simulink model "FINALBCM_Team5"  (R2018b)
settings: Solver=VariableStepAuto  SolverName=FixedStepAuto  StartTime=0.0  StopTime=4.0  RelTol=1e-3
undefined symbols (not defined in the file): sigbuilder_block
libraries: simulink x20
settings Model: Creator=99003181  LastModifiedBy=99003181
settings DataIOCC: ReturnWorkspaceOutputs=on
settings OptimizationCC: OptimizeBlockIOStorage=off  OptimizeDataStoreBuffers=off  BusAssignmentInplaceUpdate=off
settings DebuggingCC: SFUnexpectedBacktrackingDiag=warning  SFNoUnconditionalDefaultTransitionDiag=warning
settings RTWCC: GenerateReport=on  BuildConfiguration=Debug  LaunchReport=on
settings CodeAppCC: ForceParamTrailComments=on  MATLABSourceComments=on  EnableCustomComments=on
settings GRTTargetCC: CombineSignalStateStructs=on  SupportVariableSizeSignals=on  MultiInstanceErrorCode=Warning
settings ConfigComp: CovEnable=on  RecordCoverage=on  CovModelRefEnable=on

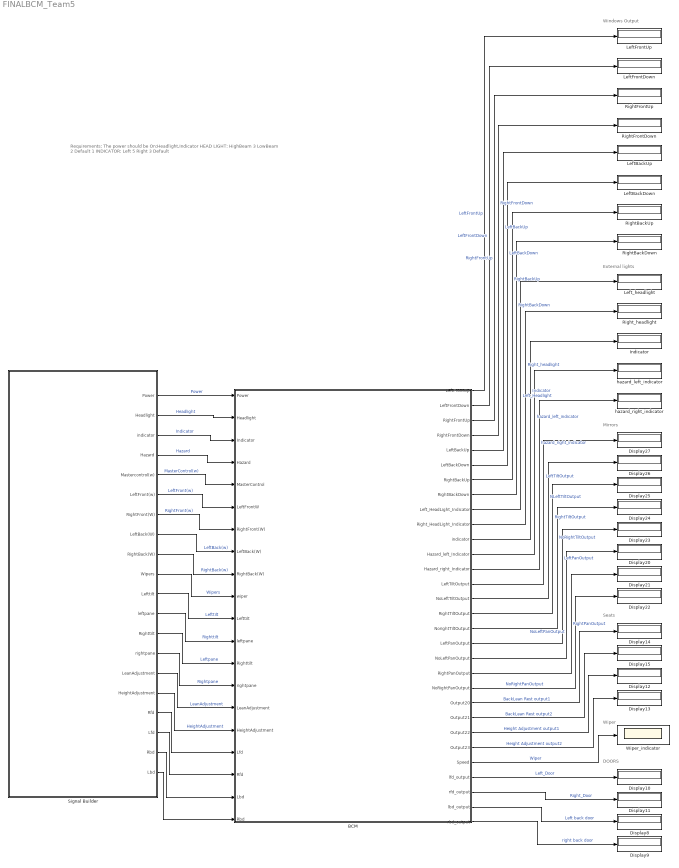
== system FINALBCM_Team5 ==
  note: Requirements:
      | The power should be On:Headlight,Indicator
      | HEAD LIGHT:
      | HighBeam	3
      | LowBeam	2
      | Default		1
      |
      | INDICATOR:
      | Left			5
      | Right 		3
      | Default
  note: Windows Output
  note: Wiper
  note: External lights
  note: Seats
  note: Mirrors
  note: DOORS
  BCM : Subsystem
  Display{8..15,20..27} (16 alike) : Display
  Indicator : Display
  LeftBackDown : Display
  LeftBackUp : Display
  LeftFrontDown : Display
  LeftFrontUp : Display
  Left_headlight : Display
  RightBackDown : Display
  RightBackUp : Display
  RightFrontDown : Display
  RightFrontUp : Display
  Right_headlight : Display
  Signal Builder : Subsystem  Tag=STV Subsys  LoadFcn=sigbuilder_block('load');  StartFcn=sigbuilder_block('start');  StopFcn=sigbuilder_block('stop');  ClipboardFcn=sigbuilder_block('clipboard');  mask(Sigbuilder block){tuvar=[0:10]}
      mask help: Simulink:masks:SigbuilderBlock_MD
      mask init:
      | if ~strcmp(get_param(bdroot(gcbh),'SimulationStatus'),'stopped') tuvar = sigbuilder_block('maskInit'); end
      settings: CopyFcn=sigbuilder_block('copy');  DeleteFcn=sigbuilder_block('delete');  ModelCloseFcn=sigbuilder_block('modelClose');  PreSaveFcn=sigbuilder_block('preSave');  PauseFcn=sigbuilder_block('pause');  ContinueFcn=sigbuilder_block('continue');  NameChangeFcn=sigbuilder_block('namechange');  OpenFcn=sigbuilder_block('open',[7.5 30.75 1011 481.5 ]);  CloseFcn=sigbuilder_block('close');
      mask Display: plot(0, 0, 100, 100,[2, 2, 32, 32, 2], [68, 8, 8, 68, 68],[32, 2], [38, 38], [32, 19, 2],[53, 60, 44], [32, 17, 17, 2],[16, 16, 31, 31]);txt = getActiveGroup(gcbh);text(2, 100, txt,'verticalAlignment', 'top');
  Wiper_indicator : Scope
  hazard_left_indicator : Display
  hazard_right_indicator : Display
  wires:
  Signal Builder/5(Mastercontrol(w)) -> BCM/5(MasterControl)  "MasterControl(w)"
  Signal Builder/8(LeftBack(W)) -> BCM/8(LeftBack(W))  "LeftBack(w)"
  Signal Builder/16(HeightAdjustment) -> BCM/16(HeightAdjustment)  "HeightAdjustment"
  Signal Builder/19(Rbd) -> BCM/19(Lbd)
  Signal Builder/11(Lefttilt) -> BCM/11(Lefttilt)  "Lefttilt"
  Signal Builder/20(Lbd) -> BCM/20(Rbd)
  Signal Builder/4(Hazard) -> BCM/4(Hazard)  "Hazard"
  Signal Builder/15(LeanAdjustment) -> BCM/15(LeanAdjustment)  "LeanAdjustment"
  Signal Builder/9(RightBack(W)) -> BCM/9(RightBack(W))  "RightBack(w)"
  Signal Builder/10(Wipers) -> BCM/10(wiper)  "Wipers"
  Signal Builder/6(LeftFront(w)) -> BCM/6(LeftFrontW)  "LeftFront(w)"
  Signal Builder/12(leftpane) -> BCM/12(leftpane)  "Righttilt"
  Signal Builder/1(Power) -> BCM/1(Power)  "Power"
  Signal Builder/7(RightFront(W)) -> BCM/7(RightFront(W))  "RightFront(w)"
  Signal Builder/14(rightpane) -> BCM/14(rightpane)  "Rightpane"
  Signal Builder/13(Righttilt) -> BCM/13(Righttilt)  "Leftpane"
  Signal Builder/2(Headlight) -> BCM/2(Headlight)  "Headlight"
  Signal Builder/17(Rfd) -> BCM/17(Lfd)
  Signal Builder/3(indicator) -> BCM/3(Indicator)  "Indicator"
  Signal Builder/18(Lfd) -> BCM/18(Rfd)
  BCM/21(NoRightPanOutput) -> Display22/1  "NoRightPanOutput"
  BCM/4(RightFrontDown) -> RightFrontDown/1  "RightFrontDown"
  BCM/12(Hazard_left_Indicator) -> hazard_left_indicator/1  "hazard_left_indicator"
  BCM/15(NoLeftTiltOutput) -> Display26/1  "NLeftTiltOutput"
  BCM/25(Output23) -> Display13/1  "Height Adjustment output2"
  BCM/26(Speed) -> Wiper_indicator/1  "Wiper"
  BCM/20(RightPanOutput) -> Display21/1  "RightPanOutput"
  BCM/1(LeftFrontUp) -> LeftFrontUp/1  "LeftFrontUp"
  BCM/24(Output22) -> Display12/1  "Height Adjustment output1"
  BCM/2(LeftFrontDown) -> LeftFrontDown/1  "LeftFrontDown"
  BCM/14(LeftTiltOutput) -> Display27/1  "LeftTiltOutput"
  BCM/10(Right_HeadLight_Indicator) -> Right_headlight/1  "Right_headlight"
  BCM/22(Output20) -> Display14/1  "BackLean Rest output1"
  BCM/7(RightBackUp) -> RightBackUp/1  "RightBackUp"
  BCM/23(Output21) -> Display15/1  "BackLean Rest output2"
  BCM/6(LeftBackDown) -> LeftBackDown/1  "LeftBackDown"
  BCM/16(RightTiltOutput) -> Display25/1  "RightTiltOutput"
  BCM/3(RightFrontUp) -> RightFrontUp/1  "RightFrontUp"
  BCM/5(LeftBackUp) -> LeftBackUp/1  "LeftBackUp"
  BCM/17(NorightTiltOutput) -> Display24/1  "NoRightTiltOutput"
  BCM/8(RightBackDown) -> RightBackDown/1  "RightBackDown"
  BCM/18(LeftPanOutput) -> Display23/1  "LeftPanOutput"
  BCM/29(lbd_output) -> Display8/1  "Left back door"
  BCM/19(NoLeftPanOutput) -> Display20/1  "NoLeftPanOutput"
  BCM/27(lfd_output) -> Display10/1  "Left_Door"
  BCM/9(Left_HeadLight_Indicator) -> Left_headlight/1  "Left_Headlight"
  BCM/30(rbd_output) -> Display9/1  "right back door"
  BCM/11(indicator) -> Indicator/1  "Indicator"
  BCM/28(rfd_output) -> Display11/1  "Right_Door"
  BCM/13(Hazard_right_Indicator) -> hazard_right_indicator/1  "hazard_right_indicator"

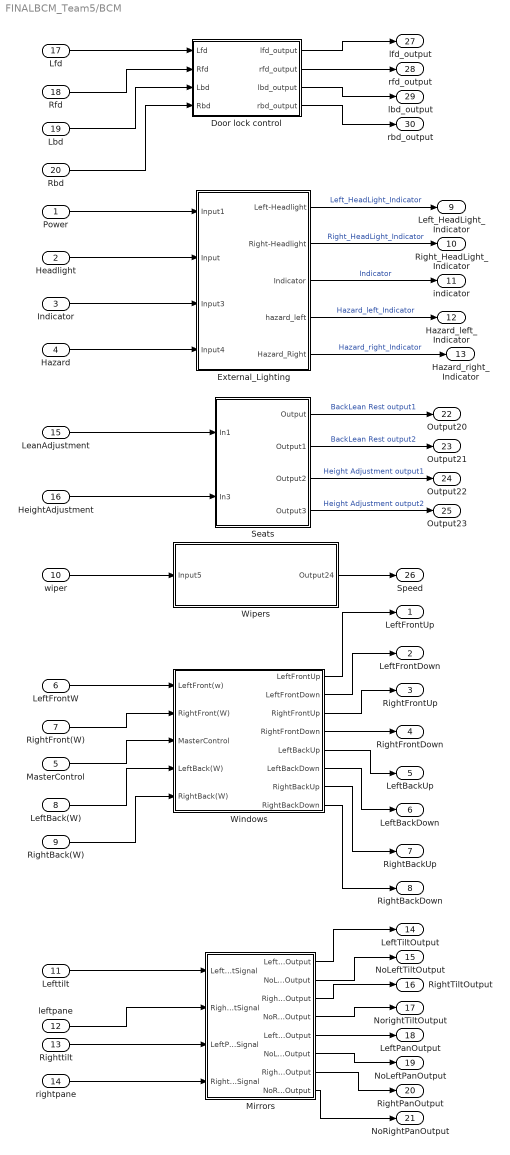
== system FINALBCM_Team5/BCM ==
  Power : Inport
  Headlight : Inport  Port=2
  Indicator : Inport  Port=3
  Hazard : Inport  Port=4
  MasterControl : Inport  Port=5
  LeftFrontW : Inport  Port=6
  RightFront(W) : Inport  Port=7
  LeftBack(W) : Inport  Port=8
  RightBack(W) : Inport  Port=9
  wiper : Inport  Port=10
  Lefttilt : Inport  Port=11
  leftpane : Inport  Port=12
  Righttilt : Inport  Port=13
  rightpane : Inport  Port=14
  LeanAdjustment : Inport  Port=15
  HeightAdjustment : Inport  Port=16
  Lfd : Inport  Port=17
  Rfd : Inport  Port=18
  Lbd : Inport  Port=19
  Rbd : Inport  Port=20
  Door lock control : Subsystem
  External_Lighting : Subsystem
  Mirrors : Subsystem
  Seats : Subsystem
  Windows : Subsystem
  Wipers : Subsystem
  LeftFrontUp : Outport
  LeftFrontDown : Outport  Port=2
  RightFrontUp : Outport  Port=3
  RightFrontDown : Outport  Port=4
  LeftBackUp : Outport  Port=5
  LeftBackDown : Outport  Port=6
  RightBackUp : Outport  Port=7
  RightBackDown : Outport  Port=8
  Left_HeadLight_Indicator : Outport  Port=9
  Right_HeadLight_Indicator : Outport  Port=10
  indicator : Outport  Port=11
  Hazard_left_Indicator : Outport  Port=12
  Hazard_right_Indicator : Outport  Port=13
  LeftTiltOutput : Outport  Port=14
  NoLeftTiltOutput : Outport  Port=15
  RightTiltOutput : Outport  Port=16
  NorightTiltOutput : Outport  Port=17
  LeftPanOutput : Outport  Port=18
  NoLeftPanOutput : Outport  Port=19
  RightPanOutput : Outport  Port=20
  NoRightPanOutput : Outport  Port=21
  Output20 : Outport  Port=22
  Output21 : Outport  Port=23
  Output22 : Outport  Port=24
  Output23 : Outport  Port=25
  Speed : Outport  Port=26
  lfd_output : Outport  Port=27
  rfd_output : Outport  Port=28
  lbd_output : Outport  Port=29
  rbd_output : Outport  Port=30
  wires:
  Seats/4("Output3 ") -> Output23/1  "Height Adjustment output2"
  LeftBack(W)/1 -> Windows/4(LeftBack(W))
  External_Lighting/5(Hazard_Right) -> Hazard_right_Indicator/1  "Hazard_right_Indicator"
  leftpane/1 -> Mirrors/2(RightTiltSignal)
  Windows/1(LeftFrontUp) -> LeftFrontUp/1
  Seats/3("Output2 ") -> Output22/1  "Height Adjustment output1"
  Windows/2(LeftFrontDown) -> LeftFrontDown/1
  wiper/1 -> Wipers/1(Input5)
  Windows/8(RightBackDown) -> RightBackDown/1
  External_Lighting/1(Left-Headlight) -> Left_HeadLight_Indicator/1  "Left_HeadLight_Indicator"
  Windows/4(RightFrontDown) -> RightFrontDown/1
  Hazard/1 -> External_Lighting/4(Input4)
  Windows/7(RightBackUp) -> RightBackUp/1
  External_Lighting/4(hazard_left) -> Hazard_left_Indicator/1  "Hazard_left_Indicator"
  Windows/3(RightFrontUp) -> RightFrontUp/1
  Windows/5(LeftBackUp) -> LeftBackUp/1
  Windows/6(LeftBackDown) -> LeftBackDown/1
  Indicator/1 -> External_Lighting/3(Input3)
  RightBack(W)/1 -> Windows/5(RightBack(W))
  Headlight/1 -> External_Lighting/2(Input)
  MasterControl/1 -> Windows/3(MasterControl)
  RightFront(W)/1 -> Windows/2(RightFront(W))
  LeftFrontW/1 -> Windows/1(LeftFront(w))
  Rfd/1 -> Door lock control/2(Rfd)
  Rbd/1 -> Door lock control/4(Rbd)
  Lbd/1 -> Door lock control/3(Lbd)
  Door lock control/4(rbd_output) -> rbd_output/1
  Door lock control/3(lbd_output) -> lbd_output/1
  Door lock control/2(rfd_output) -> rfd_output/1
  Door lock control/1(lfd_output) -> lfd_output/1
  Lfd/1 -> Door lock control/1(Lfd)
  LeanAdjustment/1 -> Seats/1("In1 ")
  Wipers/1(Output24) -> Speed/1
  External_Lighting/2(Right-Headlight) -> Right_HeadLight_Indicator/1  "Right_HeadLight_Indicator"
  Seats/1("Output ") -> Output20/1  "BackLean Rest output1"
  External_Lighting/3(Indicator) -> indicator/1  "Indicator"
  Seats/2("Output1 ") -> Output21/1  "BackLean Rest output2"
  Power/1 -> External_Lighting/1(Input1)
  HeightAdjustment/1 -> Seats/2("In3 ")
  Lefttilt/1 -> Mirrors/1(LeftTiltSignal)
  Mirrors/8(NoRightPanOutput) -> NoRightPanOutput/1
  Mirrors/7(RightPanOutput) -> RightPanOutput/1
  Mirrors/6(NoLeftPanOutput) -> NoLeftPanOutput/1
  Mirrors/5(LeftPanOutput) -> LeftPanOutput/1
  Mirrors/4(NoRightTiltOutput) -> NorightTiltOutput/1
  Mirrors/3(RightTiltOutput) -> RightTiltOutput/1
  Mirrors/2(NoLeftTiltOutput) -> NoLeftTiltOutput/1
  Mirrors/1(LeftTiltOutput) -> LeftTiltOutput/1
  rightpane/1 -> Mirrors/4(RightPanSignal)
  Righttilt/1 -> Mirrors/3(LeftPanSignal)

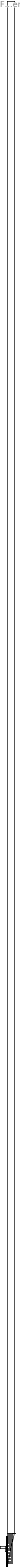
== system FINALBCM_Team5/Signal Builder ==
  Demux : Demux  Tag=STV Demux  Outputs=20
      settings: DisplayOption=none
  FromWs : FromWorkspace  Tag=STV FromWs  VariableName=tuvar
      SigBuilderData=|
      | common.afterFinalStr = 'Extrapolate'
      | common.sampleTime = 0
      | dataSet.timeRange = [0 10]
      | dataSet.name = 'Group 1'
      | sbobj.Groups.Name = 'Group 1'
      | sbobj.Groups.Signals(1).Name = 'Power'
      | sbobj.Groups.Signals(1).XData = [0 0.5 0.5 1 1 1.5 1.5 2 2 2.5 2.5 3 3 3.5 3.5 4 4.5 5 5 5.5 5.5 6 6 6.5 6.5 7 7 7.5 7.5 8 8 8.5 8.5 9 9 9.5 10]
      | sbobj.Groups.Signals(1).YData = [0.995 0.995 0 0 1 1 0 0 0.98 0.98 0 0 1 1 0 0 0 0 1 1 0 0 1 1 0 0 0.005 0.005 0 0 0.99 0.99 1 1 0 0 0]
      | sbobj.Groups.Signals(2).Name = 'Headlight'
      | sbobj.Groups.Signals(2).XData = [0 0.5 0.5 1 1 1.5 1.5 2 2 2.5 2.5 3 3 3.5 3.5 4 4 4.5 4.5 5 5 5.5 5.5 6 6 6.5 6.5 7 7 7.5 7.5 8 8 8.5 8.5 9 9 9.5 9.5 10]
      | sbobj.Groups.Signals(2).YData = [3 3 0 0 2 2 0 0 1.02 1.02 0 0 1.02 1.02 0 0 2 2 0 0 2.98 2.98 0 0 2 2 0 0 2.96 2.96 0 0 2 2 0 0 0.98 0.98 0 0]
      | sbobj.Groups.Signals(3).Name = 'indicator'
      | sbobj.Groups.Signals(3).XData = [0 0.5 0.5 1 1 1.5 1.5 2 2 2.5 2.5 3 3 3.5 3.5 4 4 4.5 4.5 5 5 5.5 5.5 6 6 6.5 6.5 7 7 7.5 7.5 8 8 8.5 8.5 9 9 9.5 9.5 10]
      | sbobj.Groups.Signals(3).YData = [5 5 0 0 0.98 0.98 0 0 3 3 0 0 5 5 0 0 3 3 0 0 2 2 0 0 1.02 1.02 0 0 1 1 0 0 -0.02 -0.02 0 0 3 3 0 0]
      | sbobj.Groups.Signals(4).Name = 'Hazard'
      | sbobj.Groups.Signals(4).XData = [0 0.5 0.5 1 1 1.5 1.5 2 2 2.5 2.5 3 3 3.5 3.5 4 4 4.5 4.5 5 5 5.5 5.5 6 6 6.5 6.5 7 7 7.5 7.5 8 8 8.5 8.5 9 9 9.5 9.5 10]
      | sbobj.Groups.Signals(4).YData = [2 2 0 0 2 2 0 0 2 2 0 0 2 2 0 0 2 2 0 0 2 2 0 0 2 2 0 0 2 2 0 0 2 2 0 0 2 2 0 0]
      | sbobj.Groups.Signals(5).Name = 'Mastercontrol(w)'
      | sbobj.Groups.Signals(5).XData = [0 1.25 1.25 6 6 9.92 9.92 10]
      | sbobj.Groups.Signals(5).YData = [0 0 1.05 1.05 0.75 0.75 0 0]
      | sbobj.Groups.Signals(6).Name = 'LeftFront(w)'
      | sbobj.Groups.Signals(6).XData = [0 2 2 3.8 3.8 10]
      | sbobj.Groups.Signals(6).YData = [0 0 1 1 -1 -1]
      | sbobj.Groups.Signals(7).Name = 'RightFront(W)'
      | sbobj.Groups.Signals(7).XData = [0 3.82 3.82 5.39 5.39 8 8 10]
      | sbobj.Groups.Signals(7).YData = [0 0 1 1 -1 -1 0.6 0.6]
      | sbobj.Groups.Signals(8).Name = 'LeftBack(W)'
      | sbobj.Groups.Signals(8).XData = [0 5.43 5.43 7.02 7.02 10]
      | sbobj.Groups.Signals(8).YData = [0 0 1 1 -1 -1]
      | sbobj.Groups.Signals(9).Name = 'RightBack(W)'
      | sbobj.Groups.Signals(9).XData = [0 7.06 7.06 8.92 8.92 10]
      | sbobj.Groups.Signals(9).YData = [0 0 1 1 -1 -1]
      | sbobj.Groups.Signals(10).Name = 'Wipers'
      | sbobj.Groups.Signals(10).XData = [0 1 1 2 2 3 3 4 4 5 5 6 6 7 7 8 8 9 9 10]
      | sbobj.Groups.Signals(10).YData = [0.2 0.2 0.4 0.4 0.6 0.6 0.2 0.2 0.4 0.4 0.6 0.6 0.2 0.2 0.4 0.4 0.6 0.6 0.2 0.2]
      | sbobj.Groups.Signals(11).Name = 'Lefttilt'
      | sbobj.Groups.Signals(11).XData = [0 3.86 3.86 5.71 5.71 10]
      | sbobj.Groups.Signals(11).YData = [0 0 1 1 0 0]
      | sbobj.Groups.Signals(12).Name = 'leftpane'
      | sbobj.Groups.Signals(12).XData = [0 2 2 3.8 3.8 10]
      | sbobj.Groups.Signals(12).YData = [0 0 1 1 0 0]
      | sbobj.Groups.Signals(13).Name = 'Righttilt'
      | sbobj.Groups.Signals(13).XData = [0 5.86 5.86 7.58 7.58 10]
      | sbobj.Groups.Signals(13).YData = [0 0 1 1 0 0]
      | sbobj.Groups.Signals(14).Name = 'rightpane'
      | sbobj.Groups.Signals(14).XData = [0 7.87 7.87 9.78 9.78 10]
      | sbobj.Groups.Signals(14).YData = [0 0 1 1 0 0]
      | sbobj.Groups.Signals(15).Name = 'LeanAdjustment'
      | sbobj.Groups.Signals(15).XData = [0 3.82 3.82 5.39 5.39 8 8 10]
      | sbobj.Groups.Signals(15).YData = [0 0 1 1 -1 -1 0.6 0.6]
      | sbobj.Groups.Signals(16).Name = 'HeightAdjustment'
      | sbobj.Groups.Signals(16).XData = [0 5.43 5.43 7.02 7.02 10]
      | sbobj.Groups.Signals(16).YData = [0 0 1 1 -1 -1]
      | sbobj.Groups.Signals(17).Name = 'Rfd'
      | sbobj.Groups.Signals(17).XData = [0 5 5 10]
      | sbobj.Groups.Signals(17).YData = [0 0 1 1]
      | sbobj.Groups.Signals(18).Name = 'Lfd'
      | sbobj.Groups.Signals(18).XData = [0 5 5 10]
      | sbobj.Groups.Signals(18).YData = [0 0 1 1]
      | sbobj.Groups.Signals(19).Name = 'Rbd'
      | sbobj.Groups.Signals(19).XData = [0 5 5 10]
      | sbobj.Groups.Signals(19).YData = [0 0 1 1]
      | sbobj.Groups.Signals(20).Name = 'Lbd'
      | sbobj.Groups.Signals(20).XData = [0 5 5 10]
      | sbobj.Groups.Signals(20).YData = [0 0 1 1]
  Power : Outport  Tag=STV Outport  VectorParamsAs1DForOutWhenUnconnected=off
  Headlight : Outport  Tag=STV Outport  Port=2  VectorParamsAs1DForOutWhenUnconnected=off
  indicator : Outport  Tag=STV Outport  Port=3  VectorParamsAs1DForOutWhenUnconnected=off
  Hazard : Outport  Tag=STV Outport  Port=4  VectorParamsAs1DForOutWhenUnconnected=off
  Mastercontrol(w) : Outport  Tag=STV Outport  Port=5
  LeftFront(w) : Outport  Tag=STV Outport  Port=6
  RightFront(W) : Outport  Tag=STV Outport  Port=7
  LeftBack(W) : Outport  Tag=STV Outport  Port=8
  RightBack(W) : Outport  Tag=STV Outport  Port=9
  Wipers : Outport  Tag=STV Outport  Port=10
  Lefttilt : Outport  Tag=STV Outport  Port=11
  leftpane : Outport  Tag=STV Outport  Port=12
  Righttilt : Outport  Tag=STV Outport  Port=13
  rightpane : Outport  Tag=STV Outport  Port=14
  LeanAdjustment : Outport  Tag=STV Outport  Port=15
  HeightAdjustment : Outport  Tag=STV Outport  Port=16
  Rfd : Outport  Tag=STV Outport  Port=17
  Lfd : Outport  Tag=STV Outport  Port=18
  Rbd : Outport  Tag=STV Outport  Port=19
  Lbd : Outport  Tag=STV Outport  Port=20
  wires:
  FromWs/1 -> Demux/1
  Demux/1 -> Power/1
  Demux/2 -> Headlight/1
  Demux/3 -> indicator/1
  Demux/4 -> Hazard/1
  Demux/5 -> Mastercontrol(w)/1
  Demux/6 -> LeftFront(w)/1
  Demux/7 -> RightFront(W)/1
  Demux/8 -> LeftBack(W)/1
  Demux/9 -> RightBack(W)/1
  Demux/10 -> Wipers/1
  Demux/11 -> Lefttilt/1
  Demux/12 -> leftpane/1
  Demux/13 -> Righttilt/1
  Demux/14 -> rightpane/1
  Demux/15 -> LeanAdjustment/1
  Demux/16 -> HeightAdjustment/1
  Demux/17 -> Rfd/1
  Demux/18 -> Lfd/1
  Demux/19 -> Rbd/1
  Demux/20 -> Lbd/1

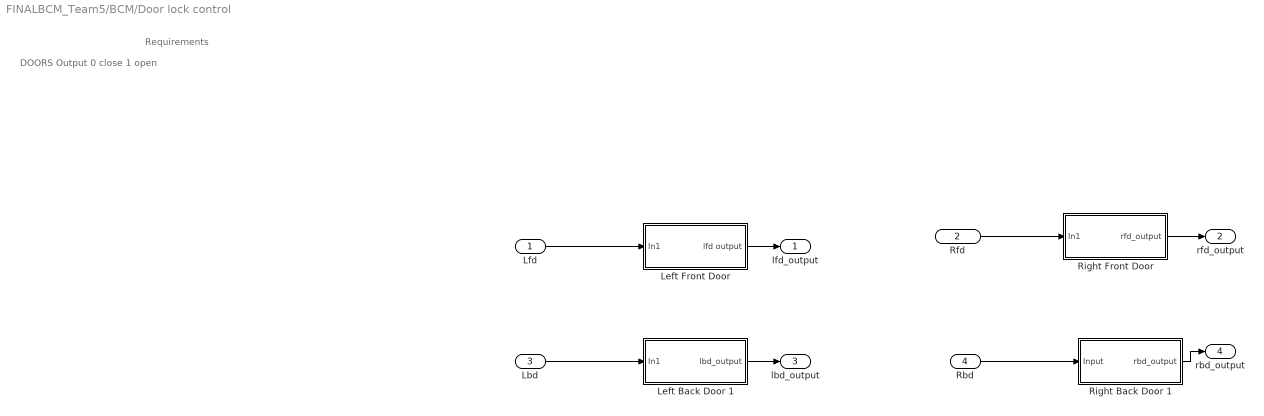
== system FINALBCM_Team5/BCM/Door lock control ==
  note: DOORS
      | Output
      |
      | 0
      | close
      |
      | 1
      | open
  note: Requirements
  Lfd : Inport
  Rfd : Inport  Port=2
  Lbd : Inport  Port=3
  Rbd : Inport  Port=4
  Left Back Door 1 : Subsystem
  "Left Front Door " : Subsystem
  Right Back Door 1 : Subsystem
  "Right Front Door " : Subsystem
  lfd_output : Outport
  rfd_output : Outport  Port=2
  lbd_output : Outport  Port=3
  rbd_output : Outport  Port=4
  wires:
  Lfd/1 -> "Left Front Door "/1(In1)
  "Left Front Door "/1(lfd output) -> lfd_output/1
  Rfd/1 -> "Right Front Door "/1(In1)
  "Right Front Door "/1(rfd_output) -> rfd_output/1
  Lbd/1 -> Left Back Door 1/1(In1)
  Left Back Door 1/1(lbd_output) -> lbd_output/1
  Rbd/1 -> Right Back Door 1/1(Input)
  Right Back Door 1/1(rbd_output) -> rbd_output/1

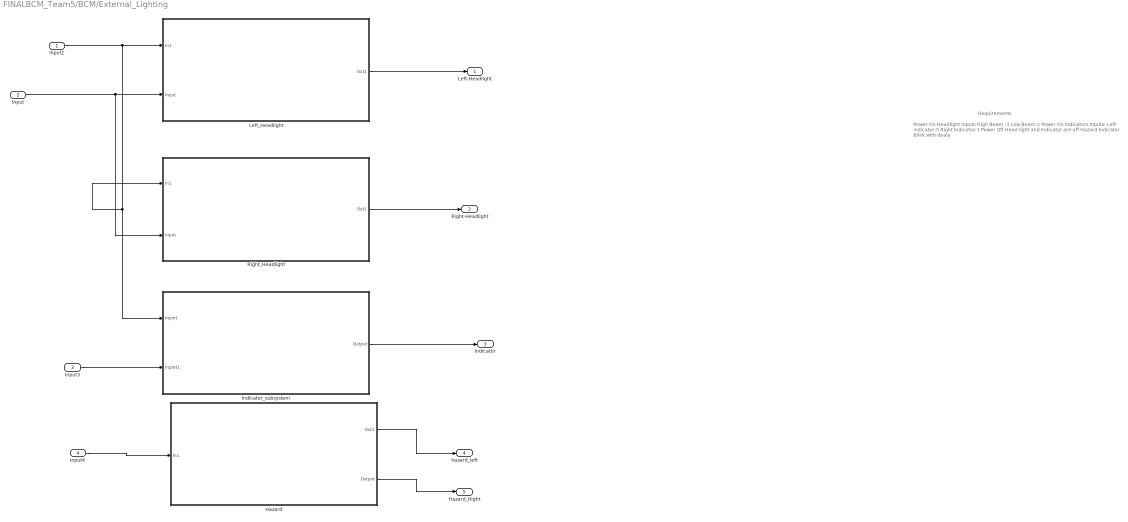
== system FINALBCM_Team5/BCM/External_Lighting ==
  note: Requirements
  note: Power
      | On
      | Headlight Inputs
      | High Beam :3
      | Low Beam:2
      |
      | Power On
      | Indicators Inputs:
      | Left indicator:5
      | Right Indicator:3
      |
      | Power Off
      | Head light and Indicator are off
      |
      | Hazard Indicator
      | Blink with dealy
  Input1 : Inport
  Input : Inport  Port=2
  Input3 : Inport  Port=3
  Input4 : Inport  Port=4
  Hazard : Subsystem
  Indicator_subsystem : Subsystem
  Left_Headlight : Subsystem
  Right_Headlight : Subsystem
  Left-Headlight : Outport  VectorParamsAs1DForOutWhenUnconnected=off
  Right-Headlight : Outport  Port=2  VectorParamsAs1DForOutWhenUnconnected=off
  Indicator : Outport  Port=3  VectorParamsAs1DForOutWhenUnconnected=off
  hazard_left : Outport  Port=4  VectorParamsAs1DForOutWhenUnconnected=off
  Hazard_Right : Outport  Port=5
  wires:
  Input1/1 -> Left_Headlight/1(In1), Indicator_subsystem/1(Inport), Right_Headlight/1(In1)
  Left_Headlight/1(Out1) -> Left-Headlight/1
  Right_Headlight/1(Out1) -> Right-Headlight/1
  Hazard/1(Out1) -> hazard_left/1
  Input4/1 -> Hazard/1(In1)
  Input/1 -> Right_Headlight/2(Input), Left_Headlight/2(Input)
  Indicator_subsystem/1(Output) -> Indicator/1
  Input3/1 -> Indicator_subsystem/2(Inport1)
  Hazard/2(Output) -> Hazard_Right/1

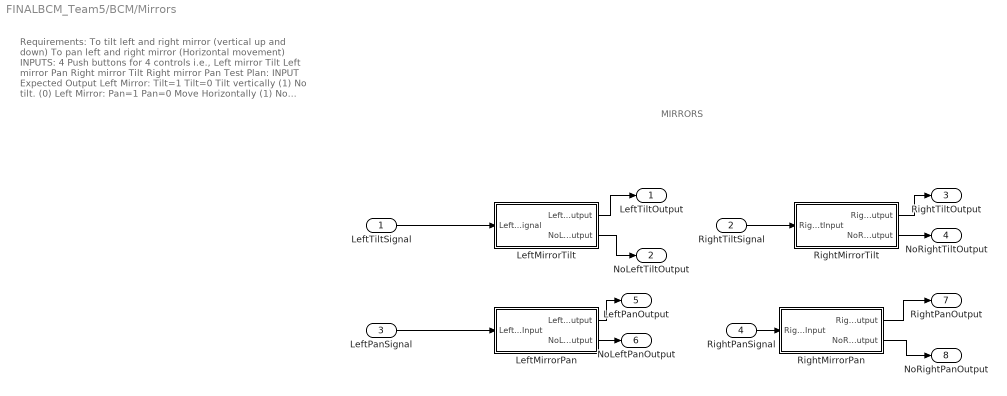
== system FINALBCM_Team5/BCM/Mirrors ==
  note: MIRRORS
  note: Requirements:
      | To tilt left and right mirror (vertical up and down)
      | To pan left and right mirror (Horizontal movement)
      | INPUTS:
      | 4 Push buttons for 4 controls i.e.,
      | Left mirror Tilt
      | Left mirror Pan
      | Right mirror Tilt
      | Right mirror Pan
      | Test Plan:
      |
      | INPUT
      | Expected Output
      |
      | Left Mirror: Tilt=1
      | Tilt=0
      | Tilt vertically (1)
      | No tilt. (0)
      |
      | Left Mirror: Pan=1
      | Pan=0
      | Move Horizontally (1)
      | No movement. (0)
      |
      | Right Mirror: Tilt=1
      | Tilt=0
      | Tilt vertically (1)
      | No tilt. (0)
      |
      | Right Mirror: Pan=1
      | Pan=0
      | Move Horizontally(1)
      | No movement.(0)
  LeftTiltSignal : Inport
  RightTiltSignal : Inport  Port=2
  LeftPanSignal : Inport  Port=3
  RightPanSignal : Inport  Port=4
  LeftMirrorPan : Subsystem
  "LeftMirrorTilt " : Subsystem
  RightMirrorPan : Subsystem
  "RightMirrorTilt " : Subsystem
  LeftTiltOutput : Outport
  NoLeftTiltOutput : Outport  Port=2
  RightTiltOutput : Outport  Port=3
  NoRightTiltOutput : Outport  Port=4
  LeftPanOutput : Outport  Port=5
  NoLeftPanOutput : Outport  Port=6
  RightPanOutput : Outport  Port=7
  NoRightPanOutput : Outport  Port=8
  wires:
  RightPanSignal/1 -> RightMirrorPan/1(RightPanInput)
  "RightMirrorTilt "/2(NoRightTiltOutput) -> NoRightTiltOutput/1
  LeftPanSignal/1 -> LeftMirrorPan/1(LeftPanInput)
  "RightMirrorTilt "/1(RightTiltOutput) -> RightTiltOutput/1
  "LeftMirrorTilt "/1(LeftTiltOutput) -> LeftTiltOutput/1
  LeftTiltSignal/1 -> "LeftMirrorTilt "/1(LeftTiltSignal)
  RightTiltSignal/1 -> "RightMirrorTilt "/1(RightTiltInput)
  LeftMirrorPan/1(LeftPanOutput) -> LeftPanOutput/1
  RightMirrorPan/1(RightPanOutput) -> RightPanOutput/1
  RightMirrorPan/2(NoRightPanOutput) -> NoRightPanOutput/1
  LeftMirrorPan/2(NoLeftPanOutput) -> NoLeftPanOutput/1
  "LeftMirrorTilt "/2(NoLeftTiltOutput) -> NoLeftTiltOutput/1

== system FINALBCM_Team5/BCM/Seats ==
  note: Requirements
      | Input
      | Output
      |
      | BackrestLean
      | 1
      | 0
      | -1
      | Invalid
      | Off
      | On
      |
      | Seatheight Adjustment
      | 1
      | 0
      | -1
      | On
      | Off
      | Invalid
  "In1 " : Inport
  "In3 " : Inport  Port=2
  BackrestLean : Subsystem
  SeatheightAdjustment : Subsystem
  "Output " : Outport
  "Output1 " : Outport  Port=2
  "Output2 " : Outport  Port=3
  "Output3 " : Outport  Port=4
  wires:
  BackrestLean/1("Output ") -> "Output "/1  "BackLean output"
  "In3 "/1 -> SeatheightAdjustment/1("In1 ")  "height input"
  SeatheightAdjustment/2("Output1 ") -> "Output3 "/1  "height output 2"
  SeatheightAdjustment/1("Output ") -> "Output2 "/1  "height Output 1"
  BackrestLean/2("Output1 ") -> "Output1 "/1  "BackLean output"
  "In1 "/1 -> BackrestLean/1("In1 ")  "BackLean Input"

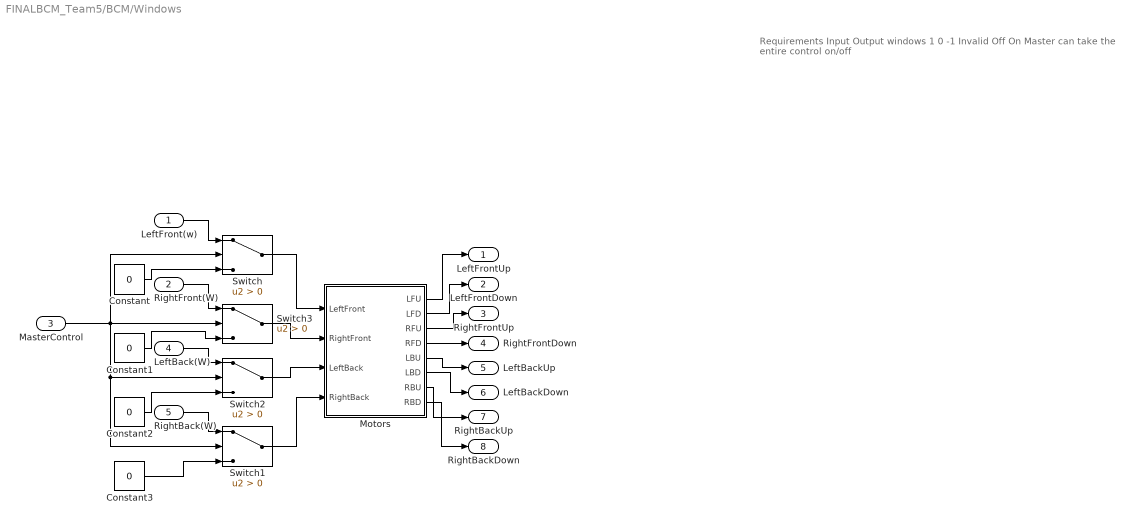
== system FINALBCM_Team5/BCM/Windows ==
  note: Requirements
      | Input
      | Output
      |
      | windows
      | 1
      | 0
      | -1
      | Invalid
      | Off
      | On
      |
      | Master
      | can take the entire control
      | on/off
  LeftFront(w) : Inport
  RightFront(W) : Inport  Port=2
  MasterControl : Inport  Port=3
  LeftBack(W) : Inport  Port=4
  RightBack(W) : Inport  Port=5
  Constant{,1..3} (4 alike) : Constant  Value=0
  Motors : Subsystem
  Switch{,1..3} (4 alike) : Switch  Criteria=u2 > Threshold
  LeftFrontUp : Outport
  LeftFrontDown : Outport  Port=2
  RightFrontUp : Outport  Port=3
  RightFrontDown : Outport  Port=4
  LeftBackUp : Outport  Port=5
  LeftBackDown : Outport  Port=6
  RightBackUp : Outport  Port=7
  RightBackDown : Outport  Port=8
  wires:
  MasterControl/1 -> Switch3/2, Switch/2, Switch1/2, Switch2/2
  Constant3/1 -> Switch1/3
  LeftBack(W)/1 -> Switch2/1
  Motors/1(LFU) -> LeftFrontUp/1
  Switch/1 -> Motors/1(LeftFront)
  LeftFront(w)/1 -> Switch/1
  Constant/1 -> Switch/3
  Switch1/1 -> Motors/4(RightBack)
  Constant2/1 -> Switch2/3
  Switch3/1 -> Motors/2(RightFront)
  Constant1/1 -> Switch3/3
  RightBack(W)/1 -> Switch1/1
  RightFront(W)/1 -> Switch3/1
  Motors/6(LBD) -> LeftBackDown/1
  Switch2/1 -> Motors/3(LeftBack)
  Motors/5(LBU) -> LeftBackUp/1
  Motors/2(LFD) -> LeftFrontDown/1
  Motors/3(RFU) -> RightFrontUp/1
  Motors/7(RBU) -> RightBackUp/1
  Motors/8(RBD) -> RightBackDown/1
  Motors/4(RFD) -> RightFrontDown/1

== system FINALBCM_Team5/BCM/Wipers ==
  note: Inputs (Sensor Input)
      | Output Speed
      |
      | Value < 10
      | Low Speed
      |
      | Value <=30
      | Mid Speed
      |
      | Value <=50
      | High Speed
      |
      | Value >50
      | Very High Speed
  Input5 : Inport
  Enable Subsystem : Subsystem  TreatAsAtomicUnit=on
  Ignition : Constant
  Subsystem : Subsystem
  scaling_factor : Gain  Gain=50
  Output24 : Outport
  wires:
  Ignition/1 -> Enable Subsystem/Enable
  Enable Subsystem/1(Out1) -> Subsystem/1(In1)
  scaling_factor/1 -> Enable Subsystem/1(In1)
  Input5/1 -> scaling_factor/1
  Subsystem/1(Out1) -> Output24/1

== system FINALBCM_Team5/BCM/Door lock control/Left Back Door 1 ==
  In1 : Inport
  Constant : Constant  Value=0
  Ramp : simulink/Sources/Ramp  slope=0  start=0  InitialOutput=1
  Switch : Switch  Criteria=u2 > Threshold
  lbd_output : Outport
  wires:
  In1/1 -> Switch/2
  Switch/1 -> lbd_output/1
  Constant/1 -> Switch/3
  Ramp/1 -> Switch/1

== system FINALBCM_Team5/BCM/Door lock control/Left Front Door  ==
  In1 : Inport
  Constant : Constant  Value=0
  Ramp : simulink/Sources/Ramp  slope=0  start=0  InitialOutput=1
  S1 : Switch  Criteria=u2 > Threshold
  lfd output : Outport
  wires:
  In1/1 -> S1/2
  S1/1 -> lfd output/1
  Constant/1 -> S1/3
  Ramp/1 -> S1/1

== system FINALBCM_Team5/BCM/Door lock control/Right Back Door 1 ==
  Input : Inport
  Constant : Constant  Value=0
  Ramp_input : simulink/Sources/Ramp  slope=0  start=0  InitialOutput=1
  Switch : Switch  Criteria=u2 > Threshold
  rbd_output : Outport
  wires:
  Input/1 -> Switch/2
  Switch/1 -> rbd_output/1
  Constant/1 -> Switch/3
  Ramp_input/1 -> Switch/1

== system FINALBCM_Team5/BCM/Door lock control/Right Front Door  ==
  In1 : Inport
  Constant : Constant  Value=0
  Ramp : simulink/Sources/Ramp  slope=0  start=0  InitialOutput=1
  Switch : Switch  Criteria=u2 > Threshold
  rfd_output : Outport
  wires:
  In1/1 -> Switch/2
  Switch/1 -> rfd_output/1
  Constant/1 -> Switch/3
  Ramp/1 -> Switch/1

== system FINALBCM_Team5/BCM/External_Lighting/Hazard ==
  In1 : Inport
  AND2 : Logic  IconShape=distinctive  AllPortsSameDT=off  OutDataTypeStr=boolean
  Enable_Input : DiscretePulseGenerator  PulseType=Time based  Period=1  PulseWidth=50
  Triggered Subsystem : Subsystem  TreatAsAtomicUnit=on
  Out1 : Outport  VectorParamsAs1DForOutWhenUnconnected=off
  Output : Outport  Port=2
  wires:
  Triggered Subsystem/1(Output) -> Output/1, Out1/1
  In1/1 -> AND2/2
  AND2/1 -> Triggered Subsystem/1(In1)
  Enable_Input/1 -> AND2/1, Triggered Subsystem/Trigger

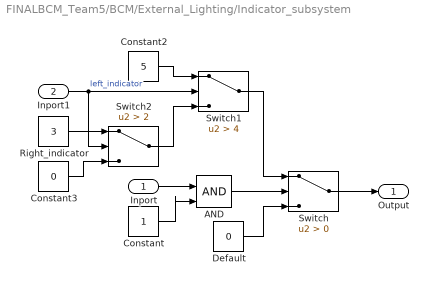
== system FINALBCM_Team5/BCM/External_Lighting/Indicator_subsystem ==
  Inport : Inport
  Inport1 : Inport  Port=2
  AND : Logic  IconShape=distinctive  AllPortsSameDT=off  OutDataTypeStr=boolean
  Constant : Constant
  Constant2 : Constant  Value=5
  Constant3 : Constant  Value=0
  Default : Constant  Value=0
  Right_indicator : Constant  Value=3
  Switch : Switch  Criteria=u2 > Threshold
  Switch1 : Switch  Criteria=u2 > Threshold  Threshold=4
  Switch2 : Switch  Criteria=u2 > Threshold  Threshold=2
  Output : Outport  VectorParamsAs1DForOutWhenUnconnected=off
  wires:
  Inport/1 -> AND/1
  Switch/1 -> Output/1
  Constant/1 -> AND/2
  Constant2/1 -> Switch1/1
  Default/1 -> Switch/3
  Switch1/1 -> Switch/1
  AND/1 -> Switch/2
  Right_indicator/1 -> Switch2/1
  Constant3/1 -> Switch2/3
  Switch2/1 -> Switch1/3
  Inport1/1 -> Switch2/2, Switch1/2  "left_indicator"

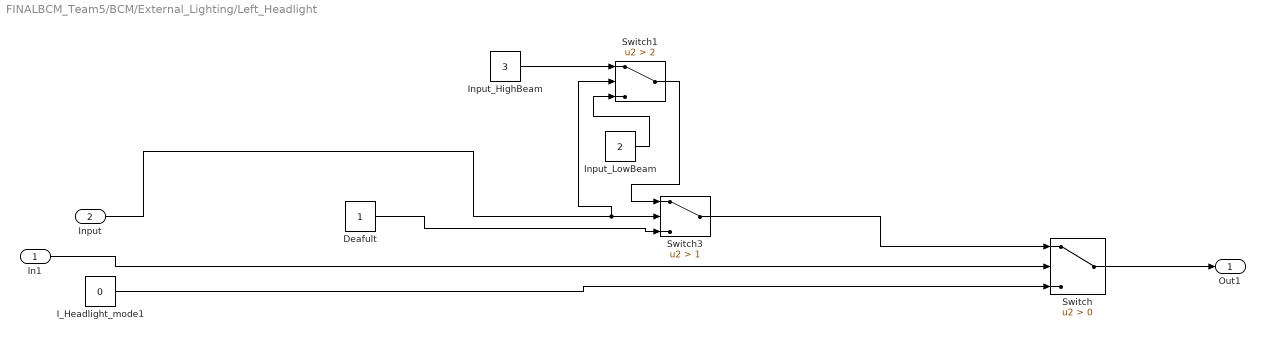
== system FINALBCM_Team5/BCM/External_Lighting/Left_Headlight ==
  In1 : Inport
  Input : Inport  Port=2
  Deafult : Constant
  I_Headlight_mode1 : Constant  Value=0
  Input_HighBeam : Constant  Value=3
  Input_LowBeam : Constant  Value=2
  Switch : Switch  Criteria=u2 > Threshold
  Switch1 : Switch  Criteria=u2 > Threshold  Threshold=2
  Switch3 : Switch  Criteria=u2 > Threshold  Threshold=1
  Out1 : Outport  VectorParamsAs1DForOutWhenUnconnected=off
  wires:
  Deafult/1 -> Switch3/3
  Input_HighBeam/1 -> Switch1/1
  Switch/1 -> Out1/1
  Input/1 -> Switch1/2, Switch3/2
  Input_LowBeam/1 -> Switch1/3
  In1/1 -> Switch/2
  I_Headlight_mode1/1 -> Switch/3
  Switch1/1 -> Switch3/1
  Switch3/1 -> Switch/1

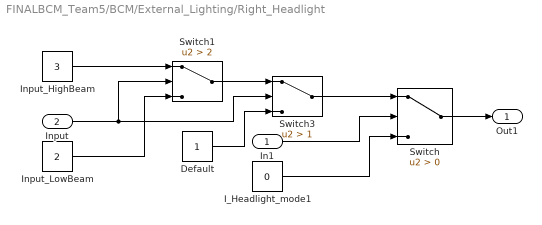
== system FINALBCM_Team5/BCM/External_Lighting/Right_Headlight ==
  In1 : Inport
  Input : Inport  Port=2
  Default : Constant
  I_Headlight_mode1 : Constant  Value=0
  Input_HighBeam : Constant  Value=3
  Input_LowBeam : Constant  Value=2
  Switch : Switch  Criteria=u2 > Threshold
  Switch1 : Switch  Criteria=u2 > Threshold  Threshold=2
  Switch3 : Switch  Criteria=u2 > Threshold  Threshold=1
  Out1 : Outport  VectorParamsAs1DForOutWhenUnconnected=off
  wires:
  Input_HighBeam/1 -> Switch1/1
  Switch/1 -> Out1/1
  I_Headlight_mode1/1 -> Switch/3
  Default/1 -> Switch3/3
  Switch3/1 -> Switch/1
  In1/1 -> Switch/2
  Input_LowBeam/1 -> Switch1/3
  Switch1/1 -> Switch3/1
  Input/1 -> Switch1/2, Switch3/2

== system FINALBCM_Team5/BCM/Mirrors/LeftMirrorPan ==
  LeftPanInput : Inport
  Constant : Constant  Value=0
  Gain : Gain  Gain=-1
  Ramp : simulink/Sources/Ramp  slope=0  start=0  InitialOutput=1
  Ramp1 : simulink/Sources/Ramp  slope=0  start=0  InitialOutput=1
  Switch : Switch  Criteria=u2 > Threshold
  Switch1 : Switch
  LeftPanOutput : Outport
  NoLeftPanOutput : Outport  Port=2
  wires:
  Ramp1/1 -> Gain/1
  LeftPanInput/1 -> Switch/2, Switch1/2
  Ramp/1 -> Switch/1
  Switch/1 -> LeftPanOutput/1
  Gain/1 -> Switch1/3
  Switch1/1 -> NoLeftPanOutput/1
  Constant/1 -> Switch1/1, Switch/3

== system FINALBCM_Team5/BCM/Mirrors/LeftMirrorTilt  ==
  LeftTiltSignal : Inport
  Constant : Constant  Value=0
  Gain : Gain  Gain=-1
  Ramp : simulink/Sources/Ramp  slope=0  start=0  InitialOutput=1
  Ramp1 : simulink/Sources/Ramp  slope=0  start=0  InitialOutput=1
  Switch : Switch  Criteria=u2 > Threshold
  Switch1 : Switch
  LeftTiltOutput : Outport
  NoLeftTiltOutput : Outport  Port=2
  wires:
  LeftTiltSignal/1 -> Switch/2, Switch1/2
  Switch/1 -> LeftTiltOutput/1  "Tilt"
  Switch1/1 -> NoLeftTiltOutput/1  "No tilt"
  Ramp1/1 -> Gain/1
  Gain/1 -> Switch1/3
  Constant/1 -> Switch1/1, Switch/3
  Ramp/1 -> Switch/1

== system FINALBCM_Team5/BCM/Mirrors/RightMirrorPan ==
  RightPanInput : Inport
  Constant : Constant  Value=0
  Gain : Gain  Gain=-1
  Ramp : simulink/Sources/Ramp  slope=0  start=0  InitialOutput=1
  Ramp1 : simulink/Sources/Ramp  slope=0  start=0  InitialOutput=1
  Switch : Switch  Criteria=u2 > Threshold
  Switch1 : Switch
  RightPanOutput : Outport
  NoRightPanOutput : Outport  Port=2
  wires:
  Ramp1/1 -> Gain/1
  RightPanInput/1 -> Switch/2, Switch1/2
  Ramp/1 -> Switch/1
  Switch/1 -> RightPanOutput/1
  Gain/1 -> Switch1/3
  Switch1/1 -> NoRightPanOutput/1
  Constant/1 -> Switch1/1, Switch/3

== system FINALBCM_Team5/BCM/Mirrors/RightMirrorTilt  ==
  RightTiltInput : Inport
  Constant : Constant  Value=0
  Gain : Gain  Gain=-1
  Ramp : simulink/Sources/Ramp  slope=0  start=0  InitialOutput=1
  Ramp1 : simulink/Sources/Ramp  slope=0  start=0  InitialOutput=1
  Switch : Switch  Criteria=u2 > Threshold
  Switch1 : Switch
  RightTiltOutput : Outport
  NoRightTiltOutput : Outport  Port=2
  wires:
  Ramp1/1 -> Gain/1
  RightTiltInput/1 -> Switch/2, Switch1/2
  Ramp/1 -> Switch/1
  Switch/1 -> RightTiltOutput/1
  Gain/1 -> Switch1/3
  Switch1/1 -> NoRightTiltOutput/1
  Constant/1 -> Switch1/1, Switch/3

== system FINALBCM_Team5/BCM/Seats/BackrestLean ==
  "In1 " : Inport
  "Constant " : Constant  Value=0
  "Gain " : Gain  Gain=-1
  "Ramp " : simulink/Sources/Ramp  slope=0  start=0  InitialOutput=1
  "Ramp1 " : simulink/Sources/Ramp  slope=0  start=0  InitialOutput=1
  "Switch " : Switch  Criteria=u2 > Threshold
  "Switch1 " : Switch
  "Output " : Outport
  "Output1 " : Outport  Port=2
  wires:
  "Ramp1 "/1 -> "Gain "/1
  "In1 "/1 -> "Switch "/2, "Switch1 "/2
  "Ramp "/1 -> "Switch "/1  "BackLean Signal"
  "Switch "/1 -> "Output "/1  "BackLean output"
  "Gain "/1 -> "Switch1 "/3
  "Switch1 "/1 -> "Output1 "/1  "BackLean Output1"
  "Constant "/1 -> "Switch1 "/1, "Switch "/3

== system FINALBCM_Team5/BCM/Seats/SeatheightAdjustment ==
  "In1 " : Inport
  "Constant " : Constant  Value=0
  "Gain " : Gain  Gain=-1
  "Ramp " : simulink/Sources/Ramp  slope=0  start=0  InitialOutput=1
  "Ramp1 " : simulink/Sources/Ramp  slope=0  start=0  InitialOutput=1
  "Switch " : Switch  Criteria=u2 > Threshold
  "Switch1 " : Switch
  "Output " : Outport
  "Output1 " : Outport  Port=2
  wires:
  "Ramp1 "/1 -> "Gain "/1
  "In1 "/1 -> "Switch "/2, "Switch1 "/2
  "Ramp "/1 -> "Switch "/1  "Height input Signal"
  "Switch "/1 -> "Output "/1  "Height output"
  "Gain "/1 -> "Switch1 "/3
  "Switch1 "/1 -> "Output1 "/1  "Height Output"
  "Constant "/1 -> "Switch1 "/1, "Switch "/3

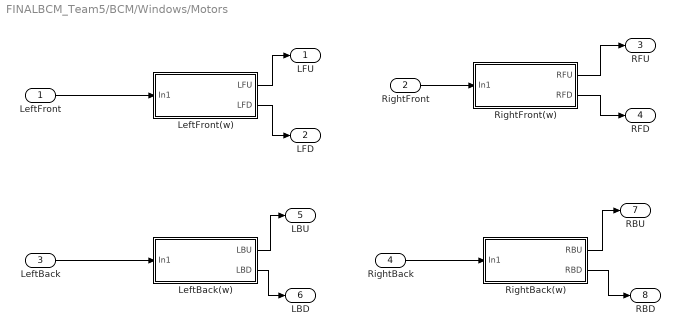
== system FINALBCM_Team5/BCM/Windows/Motors ==
  LeftFront : Inport
  RightFront : Inport  Port=2
  LeftBack : Inport  Port=3
  RightBack : Inport  Port=4
  LeftBack(w) : Subsystem
  LeftFront(w) : Subsystem
  RightBack(w) : Subsystem
  RightFront(w) : Subsystem
  LFU : Outport
  LFD : Outport  Port=2
  RFU : Outport  Port=3
  RFD : Outport  Port=4
  LBU : Outport  Port=5
  LBD : Outport  Port=6
  RBU : Outport  Port=7
  RBD : Outport  Port=8
  wires:
  LeftBack/1 -> LeftBack(w)/1(In1)
  RightFront/1 -> RightFront(w)/1(In1)
  RightBack/1 -> RightBack(w)/1(In1)
  LeftFront(w)/1(LFU) -> LFU/1
  LeftFront(w)/2(LFD) -> LFD/1
  RightFront(w)/1(RFU) -> RFU/1
  RightFront(w)/2(RFD) -> RFD/1
  RightBack(w)/1(RBU) -> RBU/1
  RightBack(w)/2(RBD) -> RBD/1
  LeftBack(w)/1(LBU) -> LBU/1
  LeftBack(w)/2(LBD) -> LBD/1
  LeftFront/1 -> LeftFront(w)/1(In1)

== system FINALBCM_Team5/BCM/Wipers/Enable Subsystem ==
  In1 : Inport
  Enable : EnablePort
  Out1 : Outport
  wires:
  In1/1 -> Out1/1

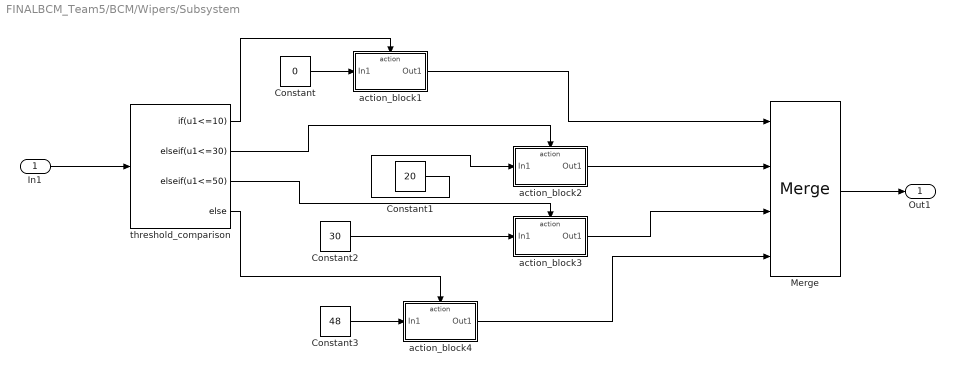
== system FINALBCM_Team5/BCM/Wipers/Subsystem ==
  In1 : Inport
  Constant : Constant  Value=0
  Constant1 : Constant  Value=20
  Constant2 : Constant  Value=30
  Constant3 : Constant  Value=48
  Merge : Merge  Inputs=4
  action_block1 : Subsystem  TreatAsAtomicUnit=on
  action_block2 : Subsystem  TreatAsAtomicUnit=on
  action_block3 : Subsystem  TreatAsAtomicUnit=on
  action_block4 : Subsystem  TreatAsAtomicUnit=on
  threshold_comparison : If  IfExpression=u1<=10  ElseIfExpressions=u1<=30,u1<=50
  Out1 : Outport
  wires:
  Constant2/1 -> action_block3/1(In1)
  action_block4/1(Out1) -> Merge/4
  Constant/1 -> action_block1/1(In1)
  threshold_comparison/3 -> action_block3/Action
  threshold_comparison/4 -> action_block4/Action
  action_block1/1(Out1) -> Merge/1
  Constant3/1 -> action_block4/1(In1)
  action_block2/1(Out1) -> Merge/2
  threshold_comparison/2 -> action_block2/Action
  threshold_comparison/1 -> action_block1/Action
  Constant1/1 -> action_block2/1(In1)
  action_block3/1(Out1) -> Merge/3
  Merge/1 -> Out1/1
  In1/1 -> threshold_comparison/1

== system FINALBCM_Team5/BCM/External_Lighting/Hazard/Triggered Subsystem ==
  In1 : Inport
  Trigger : TriggerPort  TriggerType=either  VariantControl=Variant
  Output : Outport
  wires:
  In1/1 -> Output/1

== system FINALBCM_Team5/BCM/Windows/Motors/LeftBack(w) ==
  In1 : Inport
  Constant : Constant  Value=0
  Gain : Gain  Gain=-1
  Ramp : simulink/Sources/Ramp  slope=0  start=0  InitialOutput=1
  Switch : Switch  Criteria=u2 > Threshold
  Switch1 : Switch
  LBU : Outport
  LBD : Outport  Port=2
  wires:
  Ramp/1 -> Gain/1, Switch/1
  Switch1/1 -> LBD/1
  In1/1 -> Switch/2, Switch1/2
  Switch/1 -> LBU/1
  Gain/1 -> Switch1/3
  Constant/1 -> Switch1/1, Switch/3

== system FINALBCM_Team5/BCM/Windows/Motors/LeftFront(w) ==
  In1 : Inport
  Constant : Constant  Value=0
  Gain : Gain  Gain=-1
  Ramp : simulink/Sources/Ramp  slope=0  start=0  InitialOutput=1
  Switch : Switch  Criteria=u2 > Threshold
  Switch1 : Switch
  LFU : Outport
  LFD : Outport  Port=2
  wires:
  Constant/1 -> Switch1/1, Switch/3
  In1/1 -> Switch/2, Switch1/2
  Switch/1 -> LFU/1
  Switch1/1 -> LFD/1
  Ramp/1 -> Gain/1, Switch/1
  Gain/1 -> Switch1/3

== system FINALBCM_Team5/BCM/Windows/Motors/RightBack(w) ==
  In1 : Inport
  Constant : Constant  Value=0
  Gain : Gain
  Ramp : simulink/Sources/Ramp  slope=0  start=0  InitialOutput=1
  Switch : Switch  Criteria=u2 > Threshold
  Switch1 : Switch
  RBU : Outport
  RBD : Outport  Port=2
  wires:
  Ramp/1 -> Gain/1, Switch/1
  Switch1/1 -> RBD/1
  In1/1 -> Switch/2, Switch1/2
  Switch/1 -> RBU/1
  Gain/1 -> Switch1/3
  Constant/1 -> Switch1/1, Switch/3

== system FINALBCM_Team5/BCM/Windows/Motors/RightFront(w) ==
  In1 : Inport
  Constant : Constant  Value=0
  Gain : Gain  Gain=-1
  Ramp : simulink/Sources/Ramp  slope=0  start=0  InitialOutput=1
  Switch : Switch  Criteria=u2 > Threshold
  Switch1 : Switch
  RFU : Outport
  RFD : Outport  Port=2
  wires:
  Ramp/1 -> Gain/1, Switch/1
  Switch1/1 -> RFD/1
  In1/1 -> Switch/2, Switch1/2
  Switch/1 -> RFU/1
  Gain/1 -> Switch1/3
  Constant/1 -> Switch1/1, Switch/3

== system FINALBCM_Team5/BCM/Wipers/Subsystem/action_block1 ==
  In1 : Inport
  Action Port : ActionPort
  Out1 : Outport
  wires:
  In1/1 -> Out1/1

== system FINALBCM_Team5/BCM/Wipers/Subsystem/action_block2 ==
  In1 : Inport
  Action Port : ActionPort
  Out1 : Outport
  wires:
  In1/1 -> Out1/1

== system FINALBCM_Team5/BCM/Wipers/Subsystem/action_block3 ==
  In1 : Inport
  Action Port : ActionPort
  Out1 : Outport
  wires:
  In1/1 -> Out1/1

== system FINALBCM_Team5/BCM/Wipers/Subsystem/action_block4 ==
  In1 : Inport
  Action Port : ActionPort
  Out1 : Outport
  wires:
  In1/1 -> Out1/1
